simulink model "aae364pinv2"  (Simulink 10.1)
settings: Solver=ode4  StartTime=0.0  StopTime=60  FixedStep=0.001  RelTol=1e-3  AbsTol=1e-6
values from neighbouring files (symbols this model uses):
  Beq = 5.4    [setup_ip01_2_configuration.m]
  Eff_g = 1    [setup_ip01_2_configuration.m]
  Eff_m = 1    [setup_ip01_2_configuration.m]
  g = 9.81    [setup_heli_2d_configuration.m]
  IMAX_UPM = 3    [setup_ip01_2_configuration.m]
  Kg = 3.71    [setup_ip01_2_configuration.m]
  Km = 0.804e-3 * K_RDPS2RPM    [setup_ip01_2_configuration.m]
  Kt = 1.088 * K_OZ2N * K_IN2M    [setup_ip01_2_configuration.m]
  r_mp = 0.5 / 2 * K_IN2M    [setup_ip01_2_configuration.m]
  Rm = 2.6    [setup_ip01_2_configuration.m]
  VMAX_UPM = 13    [setup_ip01_2_configuration.m]
undefined symbols (not defined in the file or in its folder): Bp, IC_ALPHA0, Ip, K, lp, Mc, Mp
libraries: simulink x1
settings Model: Creator=art  LastModifiedBy=Tomo  ExtModeArmWhenConnect=off
settings SolverCC: AutoScaleAbsTol=off
settings DataIOCC: SignalLoggingSaveFormat=ModelDataLogs
settings OptimizationCC: BooleanDataType=off  OptimizeBlockIOStorage=off  BufferReuse=off  ExpressionFolding=off  ExpressionDepthLimit=2147483647  LocalBlockOutputs=off  InitFltsAndDblsToZero=on
settings DebuggingCC: SaveWithParameterizedLinksMsg=none  SignalResolutionControl=TryResolveAllWithWarning  MultiTaskDSMMsg=warning  MultiTaskCondExecSysMsg=none  FcnCallInpInsideContextMsg=warning  StateNameClashWarn=warning
settings HardwareCC: TargetUnknown=on
settings RTWCC: SystemTargetFile=wincon.tlc  MakeCommand=make_wc  TemplateMakefile=nt_msvc.tmf
settings STFCustomTargetCC: TargetFcnLib=ansi_tfl_tmw.mat  ModelReferenceCompliant=off  CPPClassGenCompliant=on  SystemTargetFile=wincon.tlc
settings GRTTargetCC: TargetFcnLib=ansi_tfl_tmw.mat  ModelReferenceCompliant=off  ParMdlRefBuildCompliant=off  CompOptLevelCompliant=off  ConcurrentExecutionCompliant=off  MatFileLogging=off  UseToolchainInfoCompliant=off
settings CustomProperty: Value=on

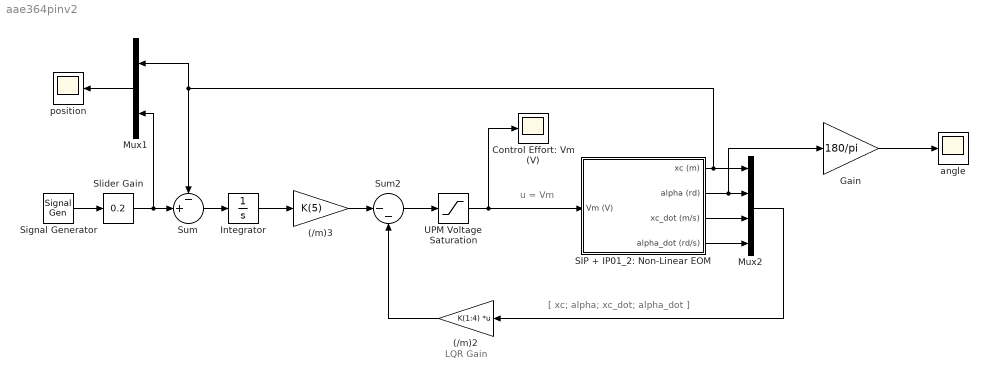
== system aae364pinv2 ==
  note: u = Vm
  note: [ xc; alpha; xc_dot; alpha_dot ]
  note: LQR Gain
  (/m)2 : Gain  Gain=K(1:4)  Multiplication=Matrix(K*u)  SaturateOnIntegerOverflow=on  OutDataTypeStr=Inherit: Same as input  ParamDataTypeStr=Inherit: Same as input
  (/m)3 : Gain  Gain=K(5)  SaturateOnIntegerOverflow=on  OutDataTypeStr=Inherit: Same as input  ParamDataTypeStr=Inherit: Same as input
  Control Effort: Vm (V) : Scope
  Gain : Gain  Gain=180/pi
  Integrator : Integrator
  Mux1 : Mux  Inputs=2
  Mux2 : Mux
  SIP + IP01_2: Non-Linear EOM : Subsystem
  Signal Generator : SignalGenerator  Frequency=1/20
  Slider Gain : simulink/Math Operations/Slider Gain  gain=0.2  low=-0.2  high=0.2
  Sum : Sum  Inputs=-+|
  Sum2 : Sum  Inputs=|--  InputSameDT=on  SaturateOnIntegerOverflow=on  OutDataTypeStr=Inherit: Same as first input
  UPM Voltage Saturation : Saturate  UpperLimit=VMAX_UPM  LowerLimit=- VMAX_UPM
  angle : Scope
  position : Scope
  wires:
  UPM Voltage Saturation/1 -> SIP + IP01_2: Non-Linear EOM/1(Vm (V)), Control Effort: Vm (V)/1
  Sum2/1 -> UPM Voltage Saturation/1
  Mux2/1 -> (/m)2/1
  (/m)2/1 -> Sum2/2
  (/m)3/1 -> Sum2/1
  SIP + IP01_2: Non-Linear EOM/1(xc (m)) -> Mux2/1, Sum/1, Mux1/1
  SIP + IP01_2: Non-Linear EOM/2(alpha (rd)) -> Mux2/2, Gain/1
  SIP + IP01_2: Non-Linear EOM/3(xc_dot (m/s)) -> Mux2/3
  SIP + IP01_2: Non-Linear EOM/4(alpha_dot (rd/s)) -> Mux2/4
  Integrator/1 -> (/m)3/1
  Sum/1 -> Integrator/1
  Slider Gain/1 -> Sum/2, Mux1/2
  Signal Generator/1 -> Slider Gain/1
  Gain/1 -> angle/1
  Mux1/1 -> position/1

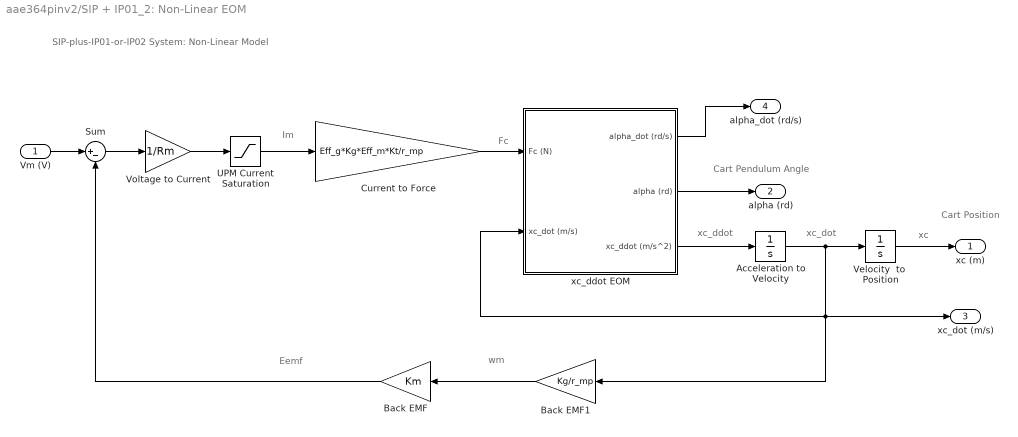
== system aae364pinv2/SIP + IP01_2: Non-Linear EOM ==
  note: SIP-plus-IP01-or-IP02 System:
      | Non-Linear Model
  note: Fc
  note: Im
  note: Eemf
  note: wm
  note: xc_dot
  note: xc_ddot
  note: xc
  note: Cart Position
  note: Cart Pendulum Angle
  Vm (V) : Inport
  Acceleration to Velocity : Integrator
  Back EMF : Gain  Gain=Km  SaturateOnIntegerOverflow=on  OutDataTypeStr=Inherit: Same as input  ParamDataTypeStr=Inherit: Same as input
  Back EMF1 : Gain  Gain=Kg/r_mp  SaturateOnIntegerOverflow=on  OutDataTypeStr=Inherit: Same as input  ParamDataTypeStr=Inherit: Same as input
  Current to Force : Gain  Gain=Eff_g*Kg*Eff_m*Kt/r_mp  SaturateOnIntegerOverflow=on  OutDataTypeStr=Inherit: Same as input  ParamDataTypeStr=Inherit: Same as input
  Sum : Sum  Inputs=|+-  InputSameDT=on  SaturateOnIntegerOverflow=on  OutDataTypeStr=Inherit: Same as first input
  "UPM Current Saturation " : Saturate  UpperLimit=IMAX_UPM  LowerLimit=- IMAX_UPM
  Velocity  to  Position : Integrator
  Voltage to Current : Gain  Gain=1/Rm  SaturateOnIntegerOverflow=on  OutDataTypeStr=Inherit: Same as input  ParamDataTypeStr=Inherit: Same as input
  xc_ddot EOM : Subsystem
  xc (m) : Outport
  alpha (rd) : Outport  Port=2
  xc_dot (m/s) : Outport  Port=3  InitialOutput=0
  alpha_dot (rd/s) : Outport  Port=4  InitialOutput=0
  wires:
  Sum/1 -> Voltage to Current/1
  Voltage to Current/1 -> "UPM Current Saturation "/1
  Acceleration to Velocity/1 -> xc_dot (m/s)/1, xc_ddot EOM/2(xc_dot (m/s)), Back EMF1/1, Velocity  to  Position/1
  Back EMF1/1 -> Back EMF/1
  Vm (V)/1 -> Sum/1
  Velocity  to  Position/1 -> xc (m)/1
  Back EMF/1 -> Sum/2
  "UPM Current Saturation "/1 -> Current to Force/1
  Current to Force/1 -> xc_ddot EOM/1(Fc (N))
  xc_ddot EOM/3(xc_ddot (m/s^2)) -> Acceleration to Velocity/1
  xc_ddot EOM/1(alpha_dot (rd/s)) -> alpha_dot (rd/s)/1
  xc_ddot EOM/2(alpha (rd)) -> alpha (rd)/1

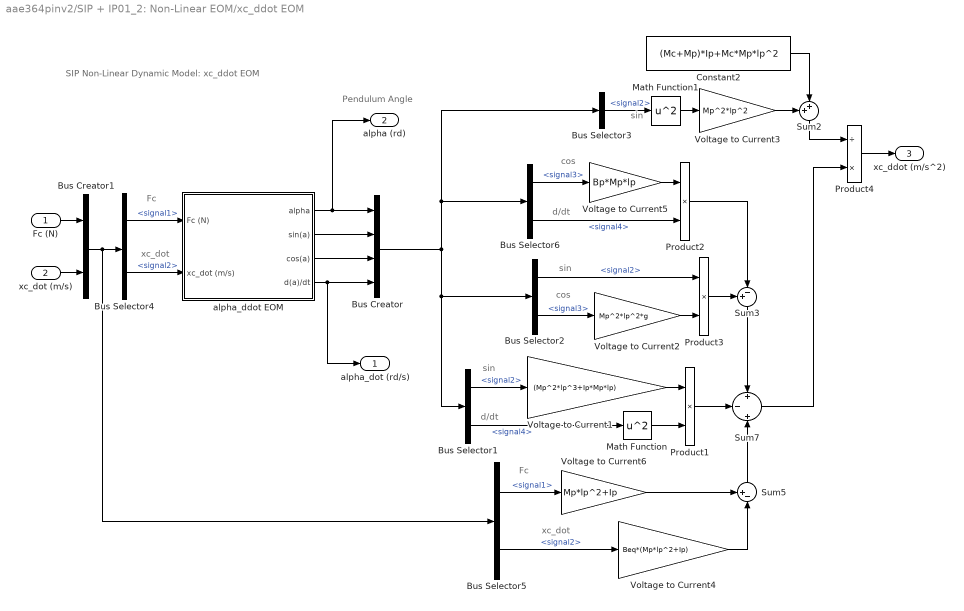
== system aae364pinv2/SIP + IP01_2: Non-Linear EOM/xc_ddot EOM ==
  note: xc_dot
  note: Fc
  note: xc_dot
  note: Fc
  note: d/dt
  note: cos
  note: Pendulum Angle
  note: sin
  note: cos
  note: sin
  note: sin
  note: d/dt
  note: SIP Non-Linear Dynamic Model:
      | xc_ddot EOM
  Fc (N) : Inport
  xc_dot (m/s) : Inport  Port=2
  Bus Creator : BusCreator  Inputs=4
  Bus Creator1 : BusCreator  Inputs=2
  Bus Selector1 : BusSelector  OutputSignals=signal2,signal4
  Bus Selector2 : BusSelector  OutputSignals=signal2,signal3
  Bus Selector3 : BusSelector  OutputSignals=signal2
  Bus Selector4 : BusSelector  OutputSignals=signal1,signal2
  Bus Selector5 : BusSelector  OutputSignals=signal1,signal2
  Bus Selector6 : BusSelector  OutputSignals=signal3,signal4
  Constant2 : Constant  Value=(Mc+Mp)*Ip+Mc*Mp*lp^2
  Math Function : Math  Operator=square  SignedPower=on  SaturateOnIntegerOverflow=on
  Math Function1 : Math  Operator=square  SignedPower=on  SaturateOnIntegerOverflow=on
  Product1 : Product  InputSameDT=on  RndMeth=Zero  SaturateOnIntegerOverflow=on  OutDataTypeStr=Inherit: Same as first input
  Product2 : Product  InputSameDT=on  RndMeth=Zero  SaturateOnIntegerOverflow=on  OutDataTypeStr=Inherit: Same as first input
  Product3 : Product  InputSameDT=on  RndMeth=Zero  SaturateOnIntegerOverflow=on  OutDataTypeStr=Inherit: Same as first input
  Product4 : Product  Inputs=/*  InputSameDT=on  RndMeth=Zero  SaturateOnIntegerOverflow=on  OutDataTypeStr=Inherit: Same as first input
  Sum2 : Sum  Inputs=++|  InputSameDT=on  SaturateOnIntegerOverflow=on  OutDataTypeStr=Inherit: Same as first input
  Sum3 : Sum  Inputs=+-|  InputSameDT=on  SaturateOnIntegerOverflow=on  OutDataTypeStr=Inherit: Same as first input
  Sum5 : Sum  Inputs=+-|  InputSameDT=on  SaturateOnIntegerOverflow=on  OutDataTypeStr=Inherit: Same as first input
  Sum7 : Sum  Inputs=+|-|+  InputSameDT=on  SaturateOnIntegerOverflow=on  OutDataTypeStr=Inherit: Same as first input
  Voltage to Current1 : Gain  Gain=(Mp^2*lp^3+Ip*Mp*lp)  SaturateOnIntegerOverflow=on  OutDataTypeStr=Inherit: Same as input  ParamDataTypeStr=Inherit: Same as input
  Voltage to Current2 : Gain  Gain=Mp^2*lp^2*g  SaturateOnIntegerOverflow=on  OutDataTypeStr=Inherit: Same as input  ParamDataTypeStr=Inherit: Same as input
  Voltage to Current3 : Gain  Gain=Mp^2*lp^2  SaturateOnIntegerOverflow=on  OutDataTypeStr=Inherit: Same as input  ParamDataTypeStr=Inherit: Same as input
  Voltage to Current4 : Gain  Gain=Beq*(Mp*lp^2+Ip)  SaturateOnIntegerOverflow=on  OutDataTypeStr=Inherit: Same as input  ParamDataTypeStr=Inherit: Same as input
  Voltage to Current5 : Gain  Gain=Bp*Mp*lp  SaturateOnIntegerOverflow=on  OutDataTypeStr=Inherit: Same as input  ParamDataTypeStr=Inherit: Same as input
  Voltage to Current6 : Gain  Gain=Mp*lp^2+Ip  SaturateOnIntegerOverflow=on  OutDataTypeStr=Inherit: Same as input  ParamDataTypeStr=Inherit: Same as input
  alpha_ddot EOM : Subsystem
  alpha_dot (rd/s) : Outport
  alpha (rd) : Outport  Port=2
  xc_ddot (m/s^2) : Outport  Port=3
  wires:
  Voltage to Current4/1 -> Sum5/2
  Voltage to Current6/1 -> Sum5/1
  Sum5/1 -> Sum7/3
  Sum3/1 -> Sum7/1
  Product3/1 -> Sum3/1
  Product2/1 -> Sum3/2
  Sum7/1 -> Product4/2
  Bus Selector5/2 -> Voltage to Current4/1  "<signal2>"
  Bus Selector5/1 -> Voltage to Current6/1  "<signal1>"
  Voltage to Current5/1 -> Product2/1
  Bus Selector2/2 -> Voltage to Current2/1  "<signal3>"
  Bus Selector2/1 -> Product3/1  "<signal2>"
  Bus Selector6/2 -> Product2/2  "<signal4>"
  Bus Selector6/1 -> Voltage to Current5/1  "<signal3>"
  Bus Selector1/1 -> Voltage to Current1/1  "<signal2>"
  Bus Selector1/2 -> Math Function/1  "<signal4>"
  Bus Selector4/2 -> alpha_ddot EOM/2(xc_dot (m/s))  "<signal2>"
  Bus Selector4/1 -> alpha_ddot EOM/1(Fc (N))  "<signal1>"
  Bus Creator1/1 -> Bus Selector5/1, Bus Selector4/1
  xc_dot (m/s)/1 -> Bus Creator1/2
  Fc (N)/1 -> Bus Creator1/1
  alpha_ddot EOM/4(d(a)/dt) -> Bus Creator/4, alpha_dot (rd/s)/1
  alpha_ddot EOM/3(cos(a)) -> Bus Creator/3
  alpha_ddot EOM/2(sin(a)) -> Bus Creator/2
  alpha_ddot EOM/1(alpha) -> alpha (rd)/1, Bus Creator/1
  Product4/1 -> xc_ddot (m/s^2)/1
  Product1/1 -> Sum7/2
  Constant2/1 -> Sum2/2
  Voltage to Current3/1 -> Sum2/1
  Math Function1/1 -> Voltage to Current3/1
  Bus Selector3/1 -> Math Function1/1  "<signal2>"
  Voltage to Current2/1 -> Product3/2
  Math Function/1 -> Product1/2
  Voltage to Current1/1 -> Product1/1
  Bus Creator/1 -> Bus Selector6/1, Bus Selector3/1, Bus Selector1/1, Bus Selector2/1
  Sum2/1 -> Product4/1

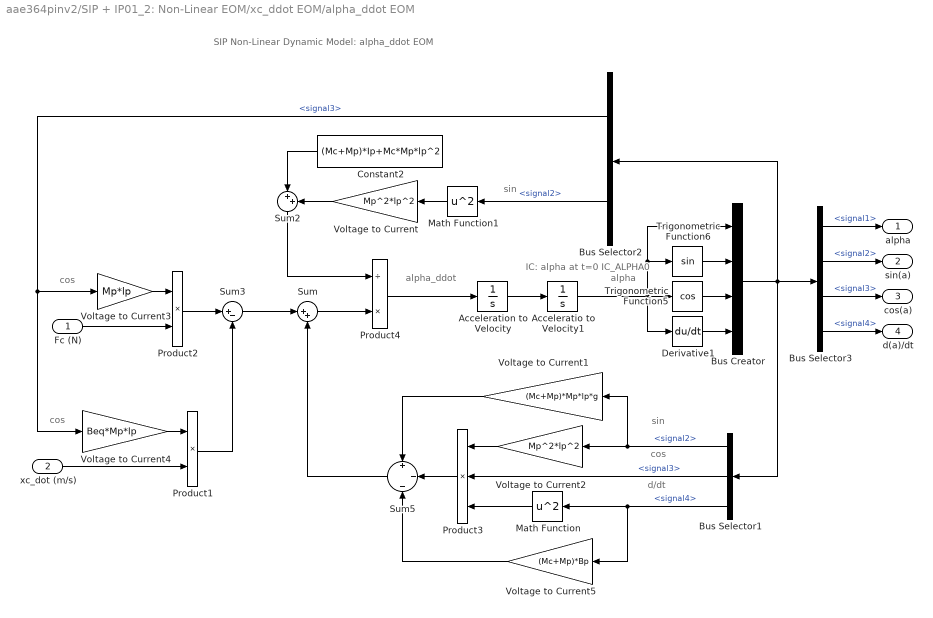
== system aae364pinv2/SIP + IP01_2: Non-Linear EOM/xc_ddot EOM/alpha_ddot EOM ==
  note: cos
  note: alpha_ddot
  note: IC: alpha at t=0
      | IC_ALPHA0
  note: SIP Non-Linear Dynamic Model:
      | alpha_ddot EOM
  note: alpha
  note: sin
  note: cos
  note: sin
  note: cos
  note: d/dt
  Fc (N) : Inport
  xc_dot (m/s) : Inport  Port=2
  Acceleratio to Velocity1 : Integrator  InitialCondition=IC_ALPHA0
  Acceleration to Velocity : Integrator
  Bus Creator : BusCreator  Inputs=4
  Bus Selector1 : BusSelector  OutputSignals=signal2,signal3,signal4
  Bus Selector2 : BusSelector  OutputSignals=signal3,signal2
  Bus Selector3 : BusSelector  OutputSignals=signal1,signal2,signal3,signal4
  Constant2 : Constant  Value=(Mc+Mp)*Ip+Mc*Mp*lp^2
  Derivative1 : Derivative
  Math Function : Math  Operator=square  SignedPower=on  SaturateOnIntegerOverflow=on
  Math Function1 : Math  Operator=square  SignedPower=on  SaturateOnIntegerOverflow=on
  Product1 : Product  InputSameDT=on  RndMeth=Zero  SaturateOnIntegerOverflow=on  OutDataTypeStr=Inherit: Same as first input
  Product2 : Product  InputSameDT=on  RndMeth=Zero  SaturateOnIntegerOverflow=on  OutDataTypeStr=Inherit: Same as first input
  Product3 : Product  Inputs=3  InputSameDT=on  RndMeth=Zero  SaturateOnIntegerOverflow=on  OutDataTypeStr=Inherit: Same as first input
  Product4 : Product  Inputs=/*  InputSameDT=on  RndMeth=Zero  SaturateOnIntegerOverflow=on  OutDataTypeStr=Inherit: Same as first input
  Sum : Sum  Inputs=|++  InputSameDT=on  SaturateOnIntegerOverflow=on  OutDataTypeStr=Inherit: Same as first input
  Sum2 : Sum  Inputs=|++  InputSameDT=on  SaturateOnIntegerOverflow=on  OutDataTypeStr=Inherit: Same as first input
  Sum3 : Sum  Inputs=|+-  InputSameDT=on  SaturateOnIntegerOverflow=on  OutDataTypeStr=Inherit: Same as first input
  Sum5 : Sum  Inputs=+|-|-  InputSameDT=on  SaturateOnIntegerOverflow=on  OutDataTypeStr=Inherit: Same as first input
  Trigonometric Function5 : Trigonometry  Operator=cos
  Trigonometric Function6 : Trigonometry
  Voltage to Current : Gain  Gain=Mp^2*lp^2  SaturateOnIntegerOverflow=on  OutDataTypeStr=Inherit: Same as input  ParamDataTypeStr=Inherit: Same as input
  Voltage to Current1 : Gain  Gain=(Mc+Mp)*Mp*lp*g  SaturateOnIntegerOverflow=on  OutDataTypeStr=Inherit: Same as input  ParamDataTypeStr=Inherit: Same as input
  Voltage to Current2 : Gain  Gain=Mp^2*lp^2  SaturateOnIntegerOverflow=on  OutDataTypeStr=Inherit: Same as input  ParamDataTypeStr=Inherit: Same as input
  Voltage to Current3 : Gain  Gain=Mp*lp  SaturateOnIntegerOverflow=on  OutDataTypeStr=Inherit: Same as input  ParamDataTypeStr=Inherit: Same as input
  Voltage to Current4 : Gain  Gain=Beq*Mp*lp  SaturateOnIntegerOverflow=on  OutDataTypeStr=Inherit: Same as input  ParamDataTypeStr=Inherit: Same as input
  Voltage to Current5 : Gain  Gain=(Mc+Mp)*Bp  SaturateOnIntegerOverflow=on  OutDataTypeStr=Inherit: Same as input  ParamDataTypeStr=Inherit: Same as input
  alpha : Outport  InitialOutput=0
  sin(a) : Outport  Port=2  InitialOutput=0
  cos(a) : Outport  Port=3  InitialOutput=0
  d(a)/dt : Outport  Port=4  InitialOutput=0
  wires:
  Sum5/1 -> Sum/2
  Voltage to Current5/1 -> Sum5/3
  Voltage to Current1/1 -> Sum5/1
  Product3/1 -> Sum5/2
  Sum3/1 -> Sum/1
  Product1/1 -> Sum3/2
  Product2/1 -> Sum3/1
  Voltage to Current4/1 -> Product1/1
  xc_dot (m/s)/1 -> Product1/2
  Fc (N)/1 -> Product2/2
  Voltage to Current3/1 -> Product2/1
  Acceleratio to Velocity1/1 -> Bus Creator/1, Trigonometric Function6/1, Derivative1/1, Trigonometric Function5/1
  Bus Selector3/4 -> d(a)/dt/1  "<signal4>"
  Bus Selector3/3 -> cos(a)/1  "<signal3>"
  Bus Selector3/2 -> sin(a)/1  "<signal2>"
  Bus Selector3/1 -> alpha/1  "<signal1>"
  Bus Selector1/3 -> Voltage to Current5/1, Math Function/1  "<signal4>"
  Bus Selector1/2 -> Product3/2  "<signal3>"
  Voltage to Current2/1 -> Product3/1
  Bus Selector2/1 -> Voltage to Current4/1, Voltage to Current3/1  "<signal3>"
  Bus Creator/1 -> Bus Selector3/1, Bus Selector1/1, Bus Selector2/1
  Derivative1/1 -> Bus Creator/4
  Trigonometric Function5/1 -> Bus Creator/3
  Trigonometric Function6/1 -> Bus Creator/2
  Constant2/1 -> Sum2/1
  Math Function1/1 -> Voltage to Current/1
  Bus Selector2/2 -> Math Function1/1  "<signal2>"
  Voltage to Current/1 -> Sum2/2
  Sum/1 -> Product4/2
  Sum2/1 -> Product4/1
  Math Function/1 -> Product3/3
  Product4/1 -> Acceleration to Velocity/1
  Bus Selector1/1 -> Voltage to Current2/1, Voltage to Current1/1  "<signal2>"
  Acceleration to Velocity/1 -> Acceleratio to Velocity1/1
